simulink model "ES259A_BattVltgCorrln"  (R2013b)
settings: Solver=FixedStepDiscrete  SolverMode=SingleTasking  StartTime=0.0  StopTime=Inf  FixedStep=0.002  RelTol=1e-3
values from neighbouring files (symbols this model uses):
  BattVltgCorrlnAllwdVltgDif = DataDict.Calibration    [ES259A_BattVltgCorrln_DataDict.m]
  BattVltgCorrlnBattLoVltg = DataDict.Calibration    [ES259A_BattVltgCorrln_DataDict.m]
  BattVltgCorrlnBattOverVltg = DataDict.Calibration    [ES259A_BattVltgCorrln_DataDict.m]
  BattVltgCorrlnBattUnderVltg = DataDict.Calibration    [ES259A_BattVltgCorrln_DataDict.m]
  BattVltgCorrlnNtc0x03C0x0440x04CFailStep = DataDict.Calibration    [ES259A_BattVltgCorrln_DataDict.m]
  BattVltgCorrlnNtc0x03C0x0440x04CPassStep = DataDict.Calibration    [ES259A_BattVltgCorrln_DataDict.m]
  BattVltgCorrlnNtc0x03DFailStep = DataDict.Calibration    [ES259A_BattVltgCorrln_DataDict.m]
  BattVltgCorrlnNtc0x03DPassStep = DataDict.Calibration    [ES259A_BattVltgCorrln_DataDict.m]
  BattVltgCorrlnNtc0x0B0FailStep = DataDict.Calibration    [ES259A_BattVltgCorrln_DataDict.m]
  BattVltgCorrlnNtc0x0B0PassStep = DataDict.Calibration    [ES259A_BattVltgCorrln_DataDict.m]
  BattVltgCorrlnNtc0x0B1FailStep = DataDict.Calibration    [ES259A_BattVltgCorrln_DataDict.m]
  BattVltgCorrlnNtc0x0B1PassStep = DataDict.Calibration    [ES259A_BattVltgCorrln_DataDict.m]
  BattVltgCorrlnNtc0x0B5FailStep = DataDict.Calibration    [ES259A_BattVltgCorrln_DataDict.m]
  BattVltgCorrlnNtc0x0B5PassStep = DataDict.Calibration    [ES259A_BattVltgCorrln_DataDict.m]
  BattVltgCorrlnRcvrlBattLoVltg = DataDict.Calibration    [ES259A_BattVltgCorrln_DataDict.m]
  BattVltgCorrlnRcvrlBattOverVltg = DataDict.Calibration    [ES259A_BattVltgCorrln_DataDict.m]
  BattVltgCorrlnRcvrlBattUnderVltg = DataDict.Calibration    [ES259A_BattVltgCorrln_DataDict.m]
  BattVltgCorrlnSysMinVltg = DataDict.ImprtdCal    [ES250A_BattVltg_DataDict.m]    (also in ES259A_BattVltgCorrln_DataDict.m = DataDict.Calibration)
  BattVltgSwdMax = DataDict.Calibration    [ES250A_BattVltg_DataDict.m]
  ELECGLBPRM_STRTUPSTPWRDISCNCTBTESTCMPL_CNT_U08 = DataDict.Constant    [ES999A_ElecGlbPrm_DataDict.m]
  SYSVLTGFLTDUALIVTR_CNT_U08 = DataDict.Constant    [ES259A_BattVltgCorrln_DataDict.m]
undefined symbols (not defined in the file or in its folder): NtcNr1, NtcSts1, SigQlfr1
libraries: simulink x14
(part 1 of 7)
settings Model: Creator=NZG49T  LastModifiedBy=nzg49t
settings SolverCC: AutoInsertRateTranBlk=on  InsertRTBMode=Always
settings DataIOCC: LimitDataPoints=off  SaveFormat=Structure  ReturnWorkspaceOutputs=on
settings OptimizationCC: BlockReduction=off  InlineParams=on  ZeroExternalMemoryAtStartup=off  ZeroInternalMemoryAtStartup=off  OptimizeModelRefInitCode=on  LifeSpan=1
settings DebuggingCC: SignalInfNanChecking=error  SignalRangeChecking=warning  UnderspecifiedInitializationDetection=Simplified  SolverPrmCheckMsg=error  InheritedTsInSrcMsg=error  DiscreteInheritContinuousMsg=error  SingleTaskRateTransMsg=error  TasksWithSamePriorityMsg=error  SigSpecEnsureSampleTimeMsg=error  CheckMatrixSingularityMsg=error  ParameterUnderflowMsg=error  ParameterPrecisionLossMsg=error  ParameterTunabilityLossMsg=error  FixptConstUnderflowMsg=warning  FixptConstOverflowMsg=warning  VectorMatrixConversionMsg=error  SignalLabelMismatchMsg=error  UnconnectedInputMsg=error  UnconnectedOutputMsg=error  UnconnectedLineMsg=error  SFcnCompatibilityMsg=error  UniqueDataStoreMsg=warning  BusObjectLabelMismatch=error  RootOutportRequireBusObject=error  AssertControl=DisableAll  ModelReferenceIOMsg=error  ModelReferenceVersionMismatchMessage=warning  ModelReferenceIOMismatchMessage=error  ModelReferenceCSMismatchMessage=warning  ModelReferenceDataLoggingMessage=error  StateNameClashWarn=warning  StrictBusMsg=ErrorOnBusTreatedAsVector  NonBusSignalsTreatedAsBus=error  SFUnexpectedBacktrackingDiag=error  SFInvalidInputDataAccessInChartInitDiag=error  SFNoUnconditionalDefaultTransitionDiag=error  SFTransitionOutsideNaturalParentDiag=error  SFUnconditionalTransitionShadowingDiag=error  SFUndirectedBroadcastEventsDiag=error
settings ModelReferenceCC: ModelReferenceNumInstancesAllowed=Single
settings RTWCC: SystemTargetFile=autosar.tlc  GenCodeOnly=on  TemplateMakefile=ert_default_tmf  Description=AUTOSAR  GenerateReport=on  ProcessScript=autosar_make_rtw_hook  LaunchReport=on
settings CodeAppCC: GenerateComments=off  IgnoreCustomStorageClasses=off  CustomSymbolStrType=$N$R$M  CustomSymbolStrBlkIO=$N$M  SimulinkBlockComments=off
settings STFCustomTargetCC: ParMdlRefBuildCompliant=on  CompOptLevelCompliant=on  IncludeMdlTerminateFcn=off  CombineOutputUpdateFcns=on  SuppressErrorStatus=on  ERTFirstTimeCompliant=on  ERTCustomFileBanners=on  SupportNonFinite=off  SupportComplex=off  SupportContinuousTime=off  SupportNonInlinedSFcns=off  MATLABClassNameForMDSCustomization=Simulink.SoftwareTarget.ERTCustomization  AutosarCompliant=on  GRTInterface=off  SystemTargetFile=autosar.tlc
settings ERTTargetCC: CodeReplacementLibrary=ANSI_C  ConcurrentExecutionCompliant=off  IncludeMdlTerminateFcn=off  SuppressErrorStatus=on  SupportNonFinite=off  SupportComplex=off  ModelStepFunctionPrototypeControlCompliant=off  CPPClassGenCompliant=off  AutosarCompliant=on  InlinedParameterPlacement=NonHierarchical  ERTCustomFileTemplate=example_file_process.tlc  EnableUserReplacementTypes=on

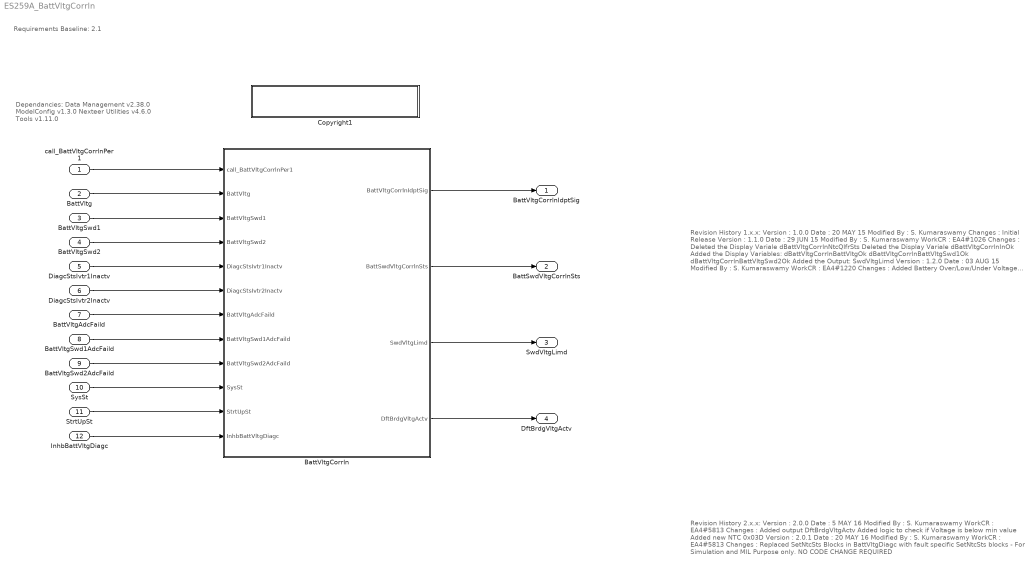
== system ES259A_BattVltgCorrln ==
  note: Revision History 1.x.x:
      |
      | Version		:	1.0.0
      | Date 		:	20 MAY 15
      | Modified By	:	S. Kumaraswamy
      | Changes		:	Initial Release
      |
      | Version		:	1.1.0
      | Date 		:	29 JUN 15
      | Modified By	:	S. Kumaraswamy
      | WorkCR 	:	EA4#1026
      | Changes		:	Deleted the Display Variale dBattVltgCorrlnNtcQlfrSts
      | 				Deleted the Display Variale dBattVltgCorrlnInOk
      | 				Added the Display Variables:
      | 					dBattVltgCorrlnBattVltgOk
      | 					dBattVltgCorrlnBattVltgSwd1Ok
      | 					dBattVltgCorrlnBattVltgSwd2Ok
      | 				Added the Output:
      | 					SwdVltgLimd
      |
      | Version		:	1.2.0
      | Date 		:	03 AUG 15
      | Modified By	:	S. Kumaraswamy
      | WorkCR 	:	EA4#1220
      | Changes		:	Added Battery Over/Low/Under Voltage Diagnostics
      | 				Added input signal InhbBattVltgDiagc
      |
      | Version		:	1.3.0
      | Date 		:	05 OCT 15
      | Modified By	:	S. Kumaraswamy
      | WorkCR 	:	EA4#1220
      | Changes		:	In .m file, InhbBattVltgDiagc.EngInit = 1 changed to InhbBattVltgDiagc.EngInit = 0
      |
      |
      | Version		:	1.4.0
      | Date 		:	18 MAR 16
      | Modified By	:	 Praveen Devaraj / Muragesh Asundi (KPIT)
      | WorkCR 	:	 EA4#4317
      | Changes		:	As per the new requirement three AdcFaild inputs and logic for these are added
      | 				The data store blocks "A" which was used for simultaion purpose  has been removed and
      |                              path where it was present earlier has been highlighted. This change has no impact on code.
  note: Dependancies:
      |
      | 	Data Management v2.38.0
      | 	ModelConfig v1.3.0
      |   	Nexteer Utilities v4.6.0
      | 	Tools v1.11.0
  note: Requirements Baseline: 2.1
  note: Revision History 2.x.x:
      |
      | Version		:	2.0.0
      | Date 		:	5 MAY 16
      | Modified By	:	S. Kumaraswamy
      | WorkCR		:	EA4#5813
      | Changes		:	Added output DftBrdgVltgActv
      | 				Added logic to check if Voltage is below min value
      | 				Added new NTC 0x03D
      |
      | Version		:	2.0.1
      | Date 		:	20 MAY 16
      | Modified By	:	S. Kumaraswamy
      | WorkCR		:	EA4#5813
      | Changes		:	Replaced SetNtcSts Blocks in BattVltgDiagc with fault specific SetNtcSts blocks - For Simulation and MIL Purpose only.
      | 				NO CODE CHANGE REQUIRED
  call_BattVltgCorrlnPer1 : Inport
  BattVltg : Inport  RequirementInfo={} %GIDa_9ae0aaec_9b84_4091_a1e8_9e8c099ef51a  Port=2
  BattVltgSwd1 : Inport  RequirementInfo={} %GIDa_9c84e353_52aa_468c_bc43_36e071f85c19  Port=3
  BattVltgSwd2 : Inport  RequirementInfo={} %GIDa_90dc59e4_2ab9_47b5_8004_0d538e7055af  Port=4
  DiagcStsIvtr1Inactv : Inport  RequirementInfo={} %GIDa_f8e15c53_514a_4131_9fe2_6d94161aaaeb  Port=5  OutDataTypeStr=boolean
  DiagcStsIvtr2Inactv : Inport  RequirementInfo={} %GIDa_3b2c6370_c505_4ccf_a518_ab0f64efa1b9  Port=6  OutDataTypeStr=boolean
  BattVltgAdcFaild : Inport  RequirementInfo={} %GIDa_ee986134_339a_4ec6_a7d6_a1f80f3bff1f  Port=7
  BattVltgSwd1AdcFaild : Inport  RequirementInfo={} %GIDa_e9391629_cfd6_4a15_93e9_ed299c660fed  Port=8
  BattVltgSwd2AdcFaild : Inport  RequirementInfo={} %GIDa_fb77af98_ead1_4424_a254_76551fbf463c  Port=9
  SysSt : Inport  RequirementInfo={} %GIDa_3959cee0_aa32_4855_b980_1d0b1d7c6b22  Port=10
  StrtUpSt : Inport  RequirementInfo={} %GIDa_35521d03_63d6_4c56_948e_5f048d51783f  Port=11
  InhbBattVltgDiagc : Inport  RequirementInfo={} %GIDa_d10198bb_1424_48c8_be8f_3c2405f9ced0  Port=12
  BattVltgCorrln : Subsystem
  Copyright1 : Subsystem  Description=|  mask(Copyright Information){none=on}
      | Copyright info block.                                               
      |                                                                     
      | Place copyright information at the top of every subsystem in design.
      mask prompts: none "No parameters"
      mask help: Place copyright information at the top of every subsystem in design.
      mask Display:
      | NxtrConf = 'Nexteer Confidential';
      | 
      | sys = bdroot; %handle for the current model ("system")
      | first = get_param(sys,'Created');
      | if(isempty(first))
      |     first = datestr(now,'yyyy');
      | else
      |     first = first(end-3:end);  %year is last four digits
      | end
      | 
      | last = get_param(sys,'LastModifiedDate');
      | if isempty(last)
      |     last = datestr(now,'yyyy');
      | else
      |     last = last(end-3:end);
      | end
      | 
      | if strcmp(first,last)
      |     fprintf('%s\nCopyright  %s Nexteer',NxtrConf,first);
      | else
      |     fprintf('%s\n%s%s-%s Nexteer',NxtrConf,char(169),first,last);
      | end
  BattVltgCorrlnIdptSig : Outport  RequirementInfo={} %GIDa_aec574ca_5fa5_4de5_85a2_6855dbe6e557
  BattSwdVltgCorrlnSts : Outport  RequirementInfo={} %GIDa_7fe09802_8610_498d_8b99_46ac352eb16c  Port=2
  SwdVltgLimd : Outport  RequirementInfo={} %GIDa_1e8b1924_aadb_4bf8_9d90_544eb8aa499f  Port=3  InitialOutput=0
  DftBrdgVltgActv : Outport  RequirementInfo={} %GIDa_446ef28e_3990_43bd_ac3d_a3cd0694cd31  Port=4  InitialOutput=0
  wires:
  BattVltgCorrln/3(SwdVltgLimd) -> SwdVltgLimd/1
  BattVltgCorrln/4(DftBrdgVltgActv) -> DftBrdgVltgActv/1
  BattVltgCorrln/2(BattSwdVltgCorrlnSts) -> BattSwdVltgCorrlnSts/1
  BattVltgCorrln/1(BattVltgCorrlnIdptSig) -> BattVltgCorrlnIdptSig/1
  BattVltgSwd2AdcFaild/1 -> BattVltgCorrln/9(BattVltgSwd2AdcFaild)
  BattVltgSwd1AdcFaild/1 -> BattVltgCorrln/8(BattVltgSwd1AdcFaild)
  SysSt/1 -> BattVltgCorrln/10(SysSt)
  StrtUpSt/1 -> BattVltgCorrln/11(StrtUpSt)
  BattVltgAdcFaild/1 -> BattVltgCorrln/7(BattVltgAdcFaild)
  InhbBattVltgDiagc/1 -> BattVltgCorrln/12(InhbBattVltgDiagc)
  DiagcStsIvtr2Inactv/1 -> BattVltgCorrln/6(DiagcStsIvtr2Inactv)
  DiagcStsIvtr1Inactv/1 -> BattVltgCorrln/5(DiagcStsIvtr1Inactv)
  BattVltgSwd2/1 -> BattVltgCorrln/4(BattVltgSwd2)
  BattVltgSwd1/1 -> BattVltgCorrln/3(BattVltgSwd1)
  BattVltg/1 -> BattVltgCorrln/2(BattVltg)
  call_BattVltgCorrlnPer1/1 -> BattVltgCorrln/1(call_BattVltgCorrlnPer1)

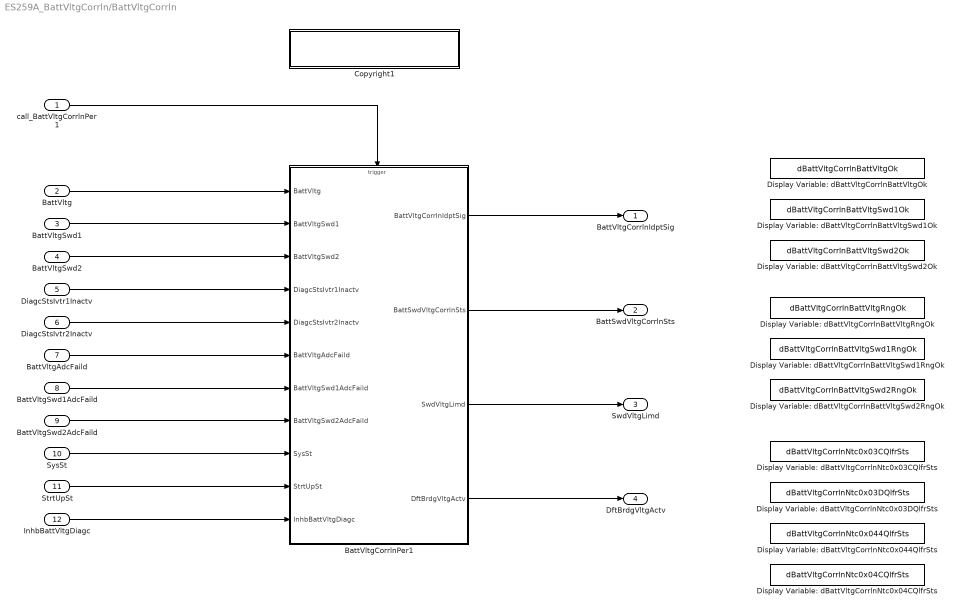
== system ES259A_BattVltgCorrln/BattVltgCorrln ==
  call_BattVltgCorrlnPer1 : Inport
  BattVltg : Inport  RequirementInfo={} %GIDa_f126ed04_401f_4bfa_94c3_1fe23454bc4c  Port=2
  BattVltgSwd1 : Inport  RequirementInfo={} %GIDa_f8722f2f_fc01_4116_8ff7_50c79c8e6a7f  Port=3
  BattVltgSwd2 : Inport  RequirementInfo={} %GIDa_5334dfc7_2389_4d4c_8517_7c435322b8bc  Port=4
  DiagcStsIvtr1Inactv : Inport  RequirementInfo={} %GIDa_58bb2539_964f_4ead_88ba_e608502c7aa6  Port=5  OutDataTypeStr=boolean
  DiagcStsIvtr2Inactv : Inport  RequirementInfo={} %GIDa_c153f17a_f8b8_4fc8_b318_6e5ea34530c6  Port=6  OutDataTypeStr=boolean
  BattVltgAdcFaild : Inport  RequirementInfo={} %GIDa_9c98f6c9_a87c_456c_aacd_351e973b6c42  Port=7
  BattVltgSwd1AdcFaild : Inport  RequirementInfo={} %GIDa_4b863112_3bcd_4930_bdb0_947e74b9095a  Port=8
  BattVltgSwd2AdcFaild : Inport  RequirementInfo={} %GIDa_42ec5868_b1c2_41ea_8fe7_d58ef520f1c8  Port=9
  SysSt : Inport  RequirementInfo={} %GIDa_f147f53a_7a4f_488c_80dd_1465aa705151  Port=10
  StrtUpSt : Inport  RequirementInfo={} %GIDa_988f5f6c_af97_4280_8e31_9d7a0d15c864  Port=11
  InhbBattVltgDiagc : Inport  RequirementInfo={} %GIDa_08e5665b_47e5_442a_9c58_120194cd1682  Port=12
  BattVltgCorrlnPer1 : Subsystem
  Copyright1 : Subsystem  Description=|  mask(Copyright Information){none=on}
      | Copyright info block.                                               
      |                                                                     
      | Place copyright information at the top of every subsystem in design.
      mask prompts: none "No parameters"
      mask help: Place copyright information at the top of every subsystem in design.
      mask Display:
      | NxtrConf = 'Nexteer Confidential';
      | 
      | sys = bdroot; %handle for the current model ("system")
      | first = get_param(sys,'Created');
      | if(isempty(first))
      |     first = datestr(now,'yyyy');
      | else
      |     first = first(end-3:end);  %year is last four digits
      | end
      | 
      | last = get_param(sys,'LastModifiedDate');
      | if isempty(last)
      |     last = datestr(now,'yyyy');
      | else
      |     last = last(end-3:end);
      | end
      | 
      | if strcmp(first,last)
      |     fprintf('%s\nCopyright  %s Nexteer',NxtrConf,first);
      | else
      |     fprintf('%s\n%s%s-%s Nexteer',NxtrConf,char(169),first,last);
      | end
  Display Variable: dBattVltgCorrlnBattVltgOk : DataStoreMemory  DataStoreName=dBattVltgCorrlnBattVltgOk  OutDataTypeStr=uint8  StateMustResolveToSignalObject=on
  Display Variable: dBattVltgCorrlnBattVltgRngOk : DataStoreMemory  DataStoreName=dBattVltgCorrlnBattVltgRngOk  OutDataTypeStr=uint8  StateMustResolveToSignalObject=on
  Display Variable: dBattVltgCorrlnBattVltgSwd1Ok : DataStoreMemory  DataStoreName=dBattVltgCorrlnBattVltgSwd1Ok  OutDataTypeStr=uint8  StateMustResolveToSignalObject=on
  Display Variable: dBattVltgCorrlnBattVltgSwd1RngOk : DataStoreMemory  DataStoreName=dBattVltgCorrlnBattVltgSwd1RngOk  OutDataTypeStr=uint8  StateMustResolveToSignalObject=on
  Display Variable: dBattVltgCorrlnBattVltgSwd2Ok : DataStoreMemory  DataStoreName=dBattVltgCorrlnBattVltgSwd2Ok  OutDataTypeStr=uint8  StateMustResolveToSignalObject=on
  Display Variable: dBattVltgCorrlnBattVltgSwd2RngOk : DataStoreMemory  DataStoreName=dBattVltgCorrlnBattVltgSwd2RngOk  OutDataTypeStr=uint8  StateMustResolveToSignalObject=on
  Display Variable: dBattVltgCorrlnNtc0x03CQlfrSts : DataStoreMemory  DataStoreName=dBattVltgCorrlnNtc0x03CQlfrSts  OutDataTypeStr=Enum: SigQlfr1  StateMustResolveToSignalObject=on
  Display Variable: dBattVltgCorrlnNtc0x03DQlfrSts : DataStoreMemory  DataStoreName=dBattVltgCorrlnNtc0x03DQlfrSts  OutDataTypeStr=Enum: SigQlfr1  StateMustResolveToSignalObject=on
  Display Variable: dBattVltgCorrlnNtc0x044QlfrSts : DataStoreMemory  DataStoreName=dBattVltgCorrlnNtc0x044QlfrSts  OutDataTypeStr=Enum: SigQlfr1  StateMustResolveToSignalObject=on
  Display Variable: dBattVltgCorrlnNtc0x04CQlfrSts : DataStoreMemory  DataStoreName=dBattVltgCorrlnNtc0x04CQlfrSts  OutDataTypeStr=Enum: SigQlfr1  StateMustResolveToSignalObject=on
  BattVltgCorrlnIdptSig : Outport  RequirementInfo={} %GIDa_5ee6736b_40f2_4c1a_b85a_65eebdb316c2
  BattSwdVltgCorrlnSts : Outport  RequirementInfo={} %GIDa_bd9620c8_c3f8_451b_a2d9_6d23915e6e1a  Port=2
  SwdVltgLimd : Outport  RequirementInfo={} %GIDa_4a11c4bf_f696_4399_ae2f_3380c1da49be  Port=3  InitialOutput=0
  DftBrdgVltgActv : Outport  RequirementInfo={} %GIDa_5c9b650e_dee9_4d60_997e_bde7a993e084  Port=4  InitialOutput=0
  wires:
  BattVltg/1 -> BattVltgCorrlnPer1/1(BattVltg)
  BattVltgSwd1/1 -> BattVltgCorrlnPer1/2(BattVltgSwd1)
  BattVltgSwd2/1 -> BattVltgCorrlnPer1/3(BattVltgSwd2)
  BattVltgCorrlnPer1/1(BattVltgCorrlnIdptSig) -> BattVltgCorrlnIdptSig/1
  DiagcStsIvtr2Inactv/1 -> BattVltgCorrlnPer1/5(DiagcStsIvtr2Inactv)
  StrtUpSt/1 -> BattVltgCorrlnPer1/10(StrtUpSt)
  SysSt/1 -> BattVltgCorrlnPer1/9(SysSt)
  DiagcStsIvtr1Inactv/1 -> BattVltgCorrlnPer1/4(DiagcStsIvtr1Inactv)
  call_BattVltgCorrlnPer1/1 -> BattVltgCorrlnPer1/Trigger
  BattVltgCorrlnPer1/2(BattSwdVltgCorrlnSts) -> BattSwdVltgCorrlnSts/1
  BattVltgCorrlnPer1/3(SwdVltgLimd) -> SwdVltgLimd/1
  InhbBattVltgDiagc/1 -> BattVltgCorrlnPer1/11(InhbBattVltgDiagc)
  BattVltgSwd2AdcFaild/1 -> BattVltgCorrlnPer1/8(BattVltgSwd2AdcFaild)
  BattVltgSwd1AdcFaild/1 -> BattVltgCorrlnPer1/7(BattVltgSwd1AdcFaild)
  BattVltgAdcFaild/1 -> BattVltgCorrlnPer1/6(BattVltgAdcFaild)
  BattVltgCorrlnPer1/4(DftBrdgVltgActv) -> DftBrdgVltgActv/1

== system ES259A_BattVltgCorrln/Copyright1 ==

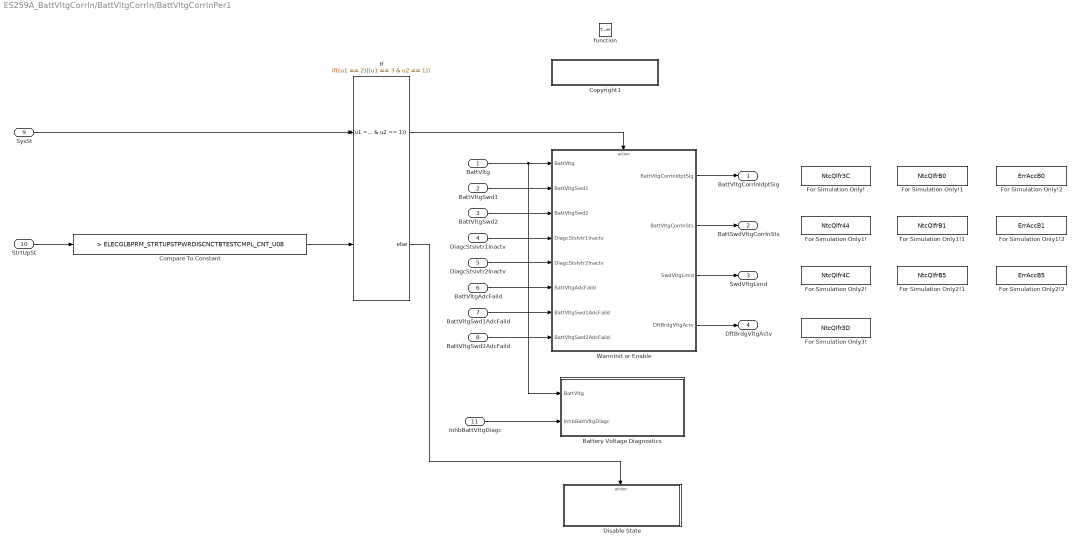
== system ES259A_BattVltgCorrln/BattVltgCorrln/BattVltgCorrlnPer1 ==
  BattVltg : Inport
  BattVltgSwd1 : Inport  Port=2  OutDataTypeStr=single
  BattVltgSwd2 : Inport  Port=3  OutDataTypeStr=single
  DiagcStsIvtr1Inactv : Inport  Port=4  OutDataTypeStr=boolean
  DiagcStsIvtr2Inactv : Inport  Port=5  OutDataTypeStr=boolean
  BattVltgAdcFaild : Inport  Port=6
  BattVltgSwd1AdcFaild : Inport  Port=7
  BattVltgSwd2AdcFaild : Inport  Port=8
  SysSt : Inport  Port=9
  StrtUpSt : Inport  Port=10
  InhbBattVltgDiagc : Inport  Port=11  OutDataTypeStr=boolean
  function : TriggerPort  TriggerType=function-call
  Battery Voltage Diagnostics : Subsystem  RequirementInfo="{'linktype_rmi_doors' '0000cf46 (/ESG Group/FDD Module Requirements/EA4 Specific/ES259A_BattVltgCorrln)' '#ES259A_171' 'true' 'REQ:  ES259A_171' '' ; 'linktype_rmi_doors' '0000cf46 (/ESG Group/FDD Module Requirements/EA4 Specific/ES259A_BattVltgCorrln)' '#ES259A_172' 'true' 'REQ:  ES259A_172' '' ; 'linktype_rmi_doors' '0000cf46 (/ESG Group/FDD Module Requirements/EA4 Specific/ES259A_BattVltgCorrln)' '#ES259A_174' 'true' 'REQ:  ES259A_174' '' ; 'linktype_rmi_doors' '0000cf46 (/ESG Group/FDD Module Requirements/EA4 Specific/ES259A_BattVltgCorrln)' '#ES259A_175' 'true' 'REQ:  ES259A_175' '' ; 'linktype_rmi_doors' '0000cf46 (/ESG Group/FDD Module Requirements/EA4 Specific/ES259A_BattVltgCorrln)' '#ES259A_177' 'true' 'REQ:  ES259A_177' '' ; 'linktype_rmi_doors' '0000cf46 (/ESG Group/FDD Module Requirements/EA4 Specific/ES259A_BattVltgCorrln)' '#ES259A_178' 'true' 'REQ:  ES259A_178' '' ; 'linktype_rmi_doors' '0000cf46 (/ESG Group/FDD Module Requirements/EA4 Specific/ES259A_BattVltgCorrln)' '#ES259A_180' 'true' 'REQ:  ES259A_180' '' ; 'linktype_rmi_doors' '0000cf46 (/ESG Group/FDD Module Requirements/EA4 Specific/ES259A_BattVltgCorrln)' '#ES259A_182' 'true' 'REQ:  ES259A_182' '' ; 'linktype_rmi_doors' '0000cf46 (/ESG Group/FDD Module Requirements/EA4 Specific/ES259A_BattVltgCorrln)' '#ES259A_183' 'true' 'REQ:  ES259A_183' '' ; 'linktype_rmi_doors' '0000cf46 (/ESG Group/FDD Module Requirements/EA4 Specific/ES259A_BattVltgCorrln)' '#ES259A_184' 'true' 'REQ:  ES259A_184' '' ; 'linktype_rmi_doors' '0000cf46 (/ESG Group/FDD Module Requirements/EA4 Specific/ES259A_BattVltgCorrln)' '#ES259A_186' 'true' 'REQ:  ES259A_186' '' ; 'linktype_rmi_doors' '0000cf46 (/ESG Group/FDD Module Requirements/EA4 Specific/ES259A_BattVltgCorrln)' '#ES259A_188' 'true' 'REQ:  ES259A_188' '' } %GIDa_c0de6c2c_8549_4a12_9f62_e9a08cdbf394"
  Compare To Constant : simulink/Logic and Bit Operations/Compare To Constant  relop=>  const=ELECGLBPRM_STRTUPSTPWRDISCNCTBTESTCMPL_CNT_U08  OutDataTypeStr=uint8
  Copyright1 : Subsystem  Description=|  mask(Copyright Information){none=on}
      | Copyright info block.                                               
      |                                                                     
      | Place copyright information at the top of every subsystem in design.
      mask prompts: none "No parameters"
      mask help: Place copyright information at the top of every subsystem in design.
      mask Display:
      | NxtrConf = 'Nexteer Confidential';
      | 
      | sys = bdroot; %handle for the current model ("system")
      | first = get_param(sys,'Created');
      | if(isempty(first))
      |     first = datestr(now,'yyyy');
      | else
      |     first = first(end-3:end);  %year is last four digits
      | end
      | 
      | last = get_param(sys,'LastModifiedDate');
      | if isempty(last)
      |     last = datestr(now,'yyyy');
      | else
      |     last = last(end-3:end);
      | end
      | 
      | if strcmp(first,last)
      |     fprintf('%s\nCopyright  %s Nexteer',NxtrConf,first);
      | else
      |     fprintf('%s\n%s%s-%s Nexteer',NxtrConf,char(169),first,last);
      | end
  Disable State : Subsystem  TreatAsAtomicUnit=on
  For Simulation Only! : DataStoreMemory  DataStoreName=NtcQlfr3C
  For Simulation Only!1 : DataStoreMemory  DataStoreName=NtcQlfrB0
  For Simulation Only!2 : DataStoreMemory  DataStoreName=ErrAccB0  OutDataTypeStr=int16
  For Simulation Only1! : DataStoreMemory  DataStoreName=NtcQlfr44
  For Simulation Only1!1 : DataStoreMemory  DataStoreName=NtcQlfrB1
  For Simulation Only1!2 : DataStoreMemory  DataStoreName=ErrAccB1  OutDataTypeStr=int16
  For Simulation Only2! : DataStoreMemory  DataStoreName=NtcQlfr4C
  For Simulation Only2!1 : DataStoreMemory  DataStoreName=NtcQlfrB5
  For Simulation Only2!2 : DataStoreMemory  DataStoreName=ErrAccB5  OutDataTypeStr=int16
  For Simulation Only3! : DataStoreMemory  DataStoreName=NtcQlfr3D
  If : If  NumInputs=2  IfExpression=(u1 == 2)|(u1 == 3 & u2 == 1)
  WarmInit or Enable : Subsystem  TreatAsAtomicUnit=on
  BattVltgCorrlnIdptSig : Outport
  BattSwdVltgCorrlnSts : Outport  RequirementInfo={} %GIDa_3ad73624_6641_44da_a28f_9988e11678b5  Port=2  InitialOutput=0
  SwdVltgLimd : Outport  RequirementInfo={} %GIDa_5f7e1f7f_e198_46a1_a24d_58ddfd5d3a89  Port=3  InitialOutput=0
  DftBrdgVltgActv : Outport  RequirementInfo={} %GIDa_cedb6ec7_b563_4bca_a7d5_9398ac57a3e7  Port=4  InitialOutput=0
  wires:
  If/2 -> Disable State/Action
  If/1 -> WarmInit or Enable/Action
  BattVltgSwd1/1 -> WarmInit or Enable/2(BattVltgSwd1)
  BattVltgSwd2/1 -> WarmInit or Enable/3(BattVltgSwd2)
  DiagcStsIvtr1Inactv/1 -> WarmInit or Enable/4(DiagcStsIvtr1Inactv)
  DiagcStsIvtr2Inactv/1 -> WarmInit or Enable/5(DiagcStsIvtr2Inactv)
  WarmInit or Enable/1(BattVltgCorrlnIdptSig) -> BattVltgCorrlnIdptSig/1
  WarmInit or Enable/2(BattVltgCorrlnSts) -> BattSwdVltgCorrlnSts/1
  StrtUpSt/1 -> Compare To Constant/1
  Compare To Constant/1 -> If/2
  SysSt/1 -> If/1
  WarmInit or Enable/3(SwdVltgLimd) -> SwdVltgLimd/1
  InhbBattVltgDiagc/1 -> Battery Voltage Diagnostics/2(InhbBattVltgDiagc)
  BattVltg/1 -> Battery Voltage Diagnostics/1(BattVltg), WarmInit or Enable/1(BattVltg)
  BattVltgAdcFaild/1 -> WarmInit or Enable/6(BattVltgAdcFaild)
  BattVltgSwd2AdcFaild/1 -> WarmInit or Enable/8(BattVltgSwd2AdcFaild)
  BattVltgSwd1AdcFaild/1 -> WarmInit or Enable/7(BattVltgSwd1AdcFaild)
  WarmInit or Enable/4(DftBrdgVltgActv) -> DftBrdgVltgActv/1

== system ES259A_BattVltgCorrln/BattVltgCorrln/Copyright1 ==

== system ES259A_BattVltgCorrln/BattVltgCorrln/BattVltgCorrlnPer1/Battery Voltage Diagnostics ==
  BattVltg : Inport
  InhbBattVltgDiagc : Inport  Port=2
  Copyright1 : Subsystem  Description=|  mask(Copyright Information){none=on}
      | Copyright info block.                                               
      |                                                                     
      | Place copyright information at the top of every subsystem in design.
      mask prompts: none "No parameters"
      mask help: Place copyright information at the top of every subsystem in design.
      mask Display:
      | NxtrConf = 'Nexteer Confidential';
      | 
      | sys = bdroot; %handle for the current model ("system")
      | first = get_param(sys,'Created');
      | if(isempty(first))
      |     first = datestr(now,'yyyy');
      | else
      |     first = first(end-3:end);  %year is last four digits
      | end
      | 
      | last = get_param(sys,'LastModifiedDate');
      | if isempty(last)
      |     last = datestr(now,'yyyy');
      | else
      |     last = last(end-3:end);
      | end
      | 
      | if strcmp(first,last)
      |     fprintf('%s\nCopyright  %s Nexteer',NxtrConf,first);
      | else
      |     fprintf('%s\n%s%s-%s Nexteer',NxtrConf,char(169),first,last);
      | end
  If : If  IfExpression=u1 == 0
  Inhibition Off : Subsystem  RequirementInfo={} %GIDa_f00050e4_548b_4aa2_8c05_f34bff13809e  TreatAsAtomicUnit=on
  Inhibition On : Subsystem  TreatAsAtomicUnit=on
  wires:
  InhbBattVltgDiagc/1 -> If/1
  If/1 -> Inhibition Off/Action
  If/2 -> Inhibition On/Action
  BattVltg/1 -> Inhibition Off/1(BattVltg)

== system ES259A_BattVltgCorrln/BattVltgCorrln/BattVltgCorrlnPer1/Copyright1 ==

== system ES259A_BattVltgCorrln/BattVltgCorrln/BattVltgCorrlnPer1/Disable State ==
  Action Port : ActionPort  ActionType=else
  Copyright1 : Subsystem  Description=|  mask(Copyright Information){none=on}
      | Copyright info block.                                               
      |                                                                     
      | Place copyright information at the top of every subsystem in design.
      mask prompts: none "No parameters"
      mask help: Place copyright information at the top of every subsystem in design.
      mask Display:
      | NxtrConf = 'Nexteer Confidential';
      | 
      | sys = bdroot; %handle for the current model ("system")
      | first = get_param(sys,'Created');
      | if(isempty(first))
      |     first = datestr(now,'yyyy');
      | else
      |     first = first(end-3:end);  %year is last four digits
      | end
      | 
      | last = get_param(sys,'LastModifiedDate');
      | if isempty(last)
      |     last = datestr(now,'yyyy');
      | else
      |     last = last(end-3:end);
      | end
      | 
      | if strcmp(first,last)
      |     fprintf('%s\nCopyright  %s Nexteer',NxtrConf,first);
      | else
      |     fprintf('%s\n%s%s-%s Nexteer',NxtrConf,char(169),first,last);
      | end

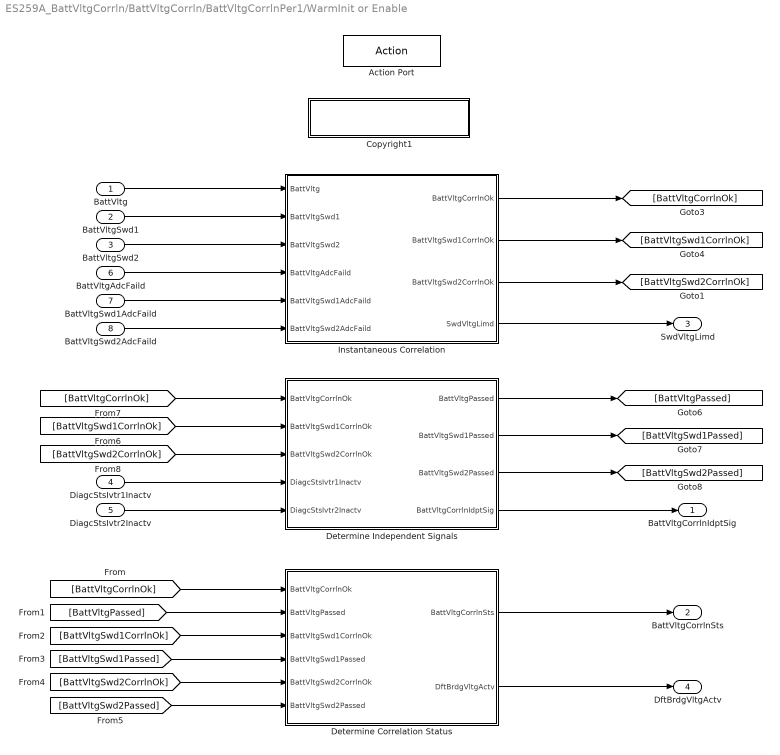
== system ES259A_BattVltgCorrln/BattVltgCorrln/BattVltgCorrlnPer1/WarmInit or Enable ==
  BattVltg : Inport
  BattVltgSwd1 : Inport  Port=2
  BattVltgSwd2 : Inport  Port=3
  DiagcStsIvtr1Inactv : Inport  RequirementInfo={} %GIDa_ea0b0d04_c797_446a_8c23_09b9fa319238  Port=4
  DiagcStsIvtr2Inactv : Inport  RequirementInfo={} %GIDa_940c0479_90c1_4645_b5ad_7886f1cabd09  Port=5
  BattVltgAdcFaild : Inport  Port=6
  BattVltgSwd1AdcFaild : Inport  Port=7
  BattVltgSwd2AdcFaild : Inport  Port=8
  Action Port : ActionPort  ActionType=then
  Copyright1 : Subsystem  Description=|  mask(Copyright Information){none=on}
      | Copyright info block.                                               
      |                                                                     
      | Place copyright information at the top of every subsystem in design.
      mask prompts: none "No parameters"
      mask help: Place copyright information at the top of every subsystem in design.
      mask Display:
      | NxtrConf = 'Nexteer Confidential';
      | 
      | sys = bdroot; %handle for the current model ("system")
      | first = get_param(sys,'Created');
      | if(isempty(first))
      |     first = datestr(now,'yyyy');
      | else
      |     first = first(end-3:end);  %year is last four digits
      | end
      | 
      | last = get_param(sys,'LastModifiedDate');
      | if isempty(last)
      |     last = datestr(now,'yyyy');
      | else
      |     last = last(end-3:end);
      | end
      | 
      | if strcmp(first,last)
      |     fprintf('%s\nCopyright  %s Nexteer',NxtrConf,first);
      | else
      |     fprintf('%s\n%s%s-%s Nexteer',NxtrConf,char(169),first,last);
      | end
  Determine Correlation Status : Subsystem  RequirementInfo="{'linktype_rmi_doors' '0000cf46 (/ESG Group/FDD Module Requirements/EA4 Specific/ES259A_BattVltgCorrln)' '#ES259A_16' 'true' 'REQ:  ES259A_16' '' ; 'linktype_rmi_doors' '0000cf46 (/ESG Group/FDD Module Requirements/EA4 Specific/ES259A_BattVltgCorrln)' '#ES259A_76' 'true' 'REQ:  ES259A_76' '' ; 'linktype_rmi_doors' '0000cf46 (/ESG Group/FDD Module Requirements/EA4 Specific/ES259A_BattVltgCorrln)' '#ES259A_75' 'true' 'REQ:  ES259A_75' '' ; 'linktype_rmi_doors' '0000cf46 (/ESG Group/FDD Module Requirements/EA4 Specific/ES259A_BattVltgCorrln)' '#ES259A_225' 'true' 'REQ:  ES259A_225' '' ; 'linktype_rmi_doors' '0000cf46 (/ESG Group/FDD Module Requirements/EA4 Specific/ES259A_BattVltgCorrln)' '#ES259A_83' 'true' 'REQ:  ES259A_83' '' ; 'linktype_rmi_doors' '0000cf46 (/ESG Group/FDD Module Requirements/EA4 Specific/ES259A_BattVltgCorrln)' '#ES259A_226' 'true' 'REQ:  ES259A_226' '' ; 'linktype_rmi_doors' '0000cf46 (/ESG Group/FDD Module Requirements/EA4 Specific/ES259A_BattVltgCorrln)' '#ES259A_84' 'true' 'REQ:  ES259A_84' '' ; 'linktype_rmi_doors' '0000cf46 (/ESG Group/FDD Module Requirements/EA4 Specific/ES259A_BattVltgCorrln)' '#ES259A_212' 'true' 'REQ:  ES259A_212' '' ; 'linktype_rmi_doors' '0000cf46 (/ESG Group/FDD Module Requirements/EA4 Specific/ES259A_BattVltgCorrln)' '#ES259A_213' 'true' 'REQ:  ES259A_213' '' } %GIDa_1d063a71_29a3_4568_848e_95b2eb318e53"  Priority=3
  Determine Independent Signals : Subsystem  RequirementInfo="{'linktype_rmi_doors' '0000cf46 (/ESG Group/FDD Module Requirements/EA4 Specific/ES259A_BattVltgCorrln)' '#ES259A_74' 'true' 'REQ:  ES259A_74' '' ; 'linktype_rmi_doors' '0000cf46 (/ESG Group/FDD Module Requirements/EA4 Specific/ES259A_BattVltgCorrln)' '#ES259A_78' 'true' 'REQ:  ES259A_78' '' ; 'linktype_rmi_doors' '0000cf46 (/ESG Group/FDD Module Requirements/EA4 Specific/ES259A_BattVltgCorrln)' '#ES259A_80' 'true' 'REQ:  ES259A_80' '' ; 'linktype_rmi_doors' '0000cf46 (/ESG Group/FDD Module Requirements/EA4 Specific/ES259A_BattVltgCorrln)' '#ES259A_73' 'true' 'REQ:  ES259A_73' '' ; 'linktype_rmi_doors' '0000cf46 (/ESG Group/FDD Module Requirements/EA4 Specific/ES259A_BattVltgCorrln)' '#ES259A_81' 'true' 'REQ:  ES259A_81' '' ; 'linktype_rmi_doors' '0000cf46 (/ESG Group/FDD Module Requirements/EA4 Specific/ES259A_BattVltgCorrln)' '#ES259A_139' 'true' 'REQ:  ES259A_139' '' ; 'linktype_rmi_doors' '0000cf46 (/ESG Group/FDD Module Requirements/EA4 Specific/ES259A_BattVltgCorrln)' '#ES259A_140' 'true' 'REQ:  ES259A_140' '' ; 'linktype_rmi_doors' '0000cf46 (/ESG Group/FDD Module Requirements/EA4 Specific/ES259A_BattVltgCorrln)' '#ES259A_141' 'true' 'REQ:  ES259A_141' '' } %GIDa_e656156f_a587_48cc_aa93_4cda59f129ee"  Priority=2
  Instantaneous Correlation : Subsystem  RequirementInfo={} %GIDa_7336d5d0_030f_4090_9dff_c7c935f04c3f  Priority=1
  BattVltgCorrlnIdptSig : Outport  RequirementInfo={} %GIDa_3db734da_8cc6_4e79_92d5_f66bd044e35c  OutDataTypeStr=uint8
  BattVltgCorrlnSts : Outport  RequirementInfo={} %GIDa_20e3ae50_7c15_4536_8fae_c5151833c420  Port=2  OutDataTypeStr=uint8
  SwdVltgLimd : Outport  RequirementInfo={} %GIDa_a517539c_da0e_494d_8ac6_5179314f6f53  Port=3  OutDataTypeStr=boolean
  DftBrdgVltgActv : Outport  Port=4
  wires:
  BattVltg/1 -> Instantaneous Correlation/1(BattVltg)
  BattVltgSwd1/1 -> Instantaneous Correlation/2(BattVltgSwd1)
  BattVltgSwd2/1 -> Instantaneous Correlation/3(BattVltgSwd2)
  Instantaneous Correlation/1(BattVltgCorrlnOk) -> [BattVltgCorrlnOk]
  Instantaneous Correlation/2(BattVltgSwd1CorrlnOk) -> [BattVltgSwd1CorrlnOk]
  [BattVltgCorrlnOk] -> Determine Independent Signals/1(BattVltgCorrlnOk)
  [BattVltgSwd1CorrlnOk] -> Determine Independent Signals/2(BattVltgSwd1CorrlnOk)
  [BattVltgSwd2CorrlnOk] -> Determine Independent Signals/3(BattVltgSwd2CorrlnOk)
  DiagcStsIvtr1Inactv/1 -> Determine Independent Signals/4(DiagcStsIvtr1Inactv)
  DiagcStsIvtr2Inactv/1 -> Determine Independent Signals/5(DiagcStsIvtr2Inactv)
  Determine Independent Signals/1(BattVltgPassed) -> [BattVltgPassed]
  Determine Independent Signals/2(BattVltgSwd1Passed) -> [BattVltgSwd1Passed]
  Determine Independent Signals/3(BattVltgSwd2Passed) -> [BattVltgSwd2Passed]
  Determine Independent Signals/4(BattVltgCorrlnIdptSig) -> BattVltgCorrlnIdptSig/1
  [BattVltgCorrlnOk] -> Determine Correlation Status/1(BattVltgCorrlnOk)
  [BattVltgPassed] -> Determine Correlation Status/2(BattVltgPassed)
  [BattVltgSwd1CorrlnOk] -> Determine Correlation Status/3(BattVltgSwd1CorrlnOk)
  [BattVltgSwd1Passed] -> Determine Correlation Status/4(BattVltgSwd1Passed)
  [BattVltgSwd2CorrlnOk] -> Determine Correlation Status/5(BattVltgSwd2CorrlnOk)
  [BattVltgSwd2Passed] -> Determine Correlation Status/6(BattVltgSwd2Passed)
  Determine Correlation Status/1(BattVltgCorrlnSts) -> BattVltgCorrlnSts/1
  Instantaneous Correlation/4(SwdVltgLimd) -> SwdVltgLimd/1
  BattVltgAdcFaild/1 -> Instantaneous Correlation/4(BattVltgAdcFaild)
  BattVltgSwd1AdcFaild/1 -> Instantaneous Correlation/5(BattVltgSwd1AdcFaild)
  BattVltgSwd2AdcFaild/1 -> Instantaneous Correlation/6(BattVltgSwd2AdcFaild)
  Determine Correlation Status/2(DftBrdgVltgActv) -> DftBrdgVltgActv/1
  Instantaneous Correlation/3(BattVltgSwd2CorrlnOk) -> [BattVltgSwd2CorrlnOk]

== system ES259A_BattVltgCorrln/BattVltgCorrln/BattVltgCorrlnPer1/Battery Voltage Diagnostics/Copyright1 ==

== system ES259A_BattVltgCorrln/BattVltgCorrln/BattVltgCorrlnPer1/Battery Voltage Diagnostics/Inhibition Off ==
  note: Outside Operational Voltage Range (No Assist)						0x0B0
      | 	Under Minimum Battery Voltage
      | Extended Voltage Range, Low Voltage (Extended Performance)			0x0B1
      | 	Low Battery Voltage
      | Outside Operational Voltage Range (No Assist)						0x0B5
      | 	Over Maximum Battery Voltage
  BattVltg : Inport
  Action Port : ActionPort  ActionType=then
  BattVltg < UnderVltg : Subsystem  RequirementInfo={} %GIDa_27210ad8_0da4_4b7d_ad34_47372fdcd46e  TreatAsAtomicUnit=on
  BattVltg > OverVltg : Subsystem  RequirementInfo={} %GIDa_f678b1bc_f111_4fcf_b4f9_eeaa0479fbc9  TreatAsAtomicUnit=on
  Constant : Constant  Value=BattVltgCorrlnBattLoVltg
  Constant1 : Constant  Value=BattVltgCorrlnBattOverVltg
  Constant2 : Constant  Value=BattVltgCorrlnBattUnderVltg
  Copyright1 : Subsystem  Description=|  mask(Copyright Information){none=on}
      | Copyright info block.                                               
      |                                                                     
      | Place copyright information at the top of every subsystem in design.
      mask prompts: none "No parameters"
      mask help: Place copyright information at the top of every subsystem in design.
      mask Display:
      | NxtrConf = 'Nexteer Confidential';
      | 
      | sys = bdroot; %handle for the current model ("system")
      | first = get_param(sys,'Created');
      | if(isempty(first))
      |     first = datestr(now,'yyyy');
      | else
      |     first = first(end-3:end);  %year is last four digits
      | end
      | 
      | last = get_param(sys,'LastModifiedDate');
      | if isempty(last)
      |     last = datestr(now,'yyyy');
      | else
      |     last = last(end-3:end);
      | end
      | 
      | if strcmp(first,last)
      |     fprintf('%s\nCopyright  %s Nexteer',NxtrConf,first);
      | else
      |     fprintf('%s\n%s%s-%s Nexteer',NxtrConf,char(169),first,last);
      | end
  If : If  NumInputs=4  IfExpression=u1 > u2  ElseIfExpressions=((u1 < u3) & (u1 >= u4)), u1 < u4
  LowVltg <= Batt <= OverVltg : Subsystem  RequirementInfo={} %GIDa_9c974e7b_bca6_4d23_a789_0c8532e06c78  TreatAsAtomicUnit=on
  UnderVltg <= BattVltg < LowVltg : Subsystem  RequirementInfo={} %GIDa_4ff1a3e6_7cb5_4c5b_8a30_2a844fcdd7f9  TreatAsAtomicUnit=on
  wires:
  Constant1/1 -> If/2
  Constant2/1 -> If/4
  Constant/1 -> If/3
  If/1 -> BattVltg > OverVltg/Action
  If/2 -> UnderVltg <= BattVltg < LowVltg/Action
  If/3 -> BattVltg < UnderVltg/Action
  If/4 -> LowVltg <= Batt <= OverVltg/Action
  BattVltg/1 -> UnderVltg <= BattVltg < LowVltg/1(BattVltg), LowVltg <= Batt <= OverVltg/1(BattVltg), If/1

== system ES259A_BattVltgCorrln/BattVltgCorrln/BattVltgCorrlnPer1/Battery Voltage Diagnostics/Inhibition On ==
  Action Port : ActionPort  ActionType=else
  Copyright1 : Subsystem  Description=|  mask(Copyright Information){none=on}
      | Copyright info block.                                               
      |                                                                     
      | Place copyright information at the top of every subsystem in design.
      mask prompts: none "No parameters"
      mask help: Place copyright information at the top of every subsystem in design.
      mask Display:
      | NxtrConf = 'Nexteer Confidential';
      | 
      | sys = bdroot; %handle for the current model ("system")
      | first = get_param(sys,'Created');
      | if(isempty(first))
      |     first = datestr(now,'yyyy');
      | else
      |     first = first(end-3:end);  %year is last four digits
      | end
      | 
      | last = get_param(sys,'LastModifiedDate');
      | if isempty(last)
      |     last = datestr(now,'yyyy');
      | else
      |     last = last(end-3:end);
      | end
      | 
      | if strcmp(first,last)
      |     fprintf('%s\nCopyright  %s Nexteer',NxtrConf,first);
      | else
      |     fprintf('%s\n%s%s-%s Nexteer',NxtrConf,char(169),first,last);
      | end

== system ES259A_BattVltgCorrln/BattVltgCorrln/BattVltgCorrlnPer1/Disable State/Copyright1 ==

== system ES259A_BattVltgCorrln/BattVltgCorrln/BattVltgCorrlnPer1/WarmInit or Enable/Copyright1 ==

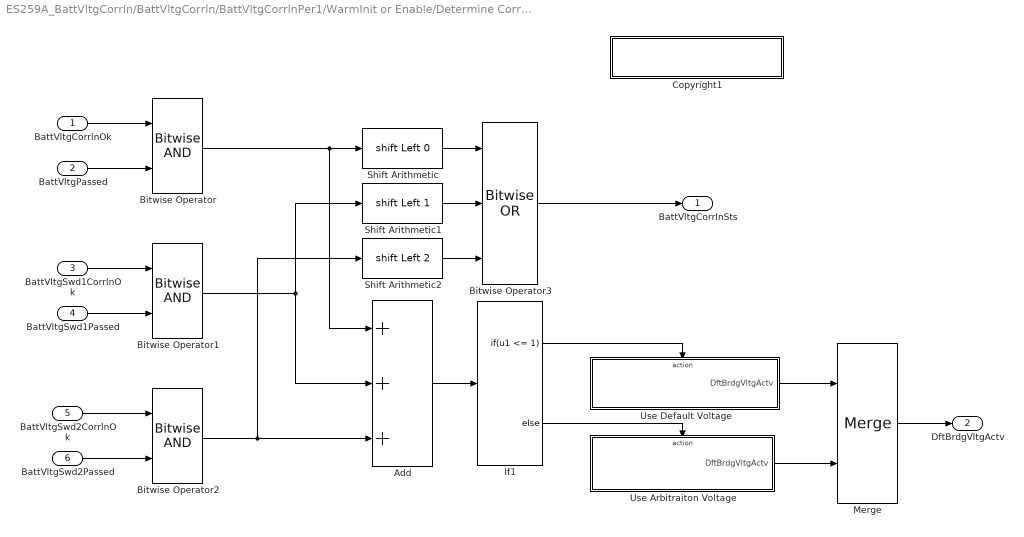
== system ES259A_BattVltgCorrln/BattVltgCorrln/BattVltgCorrlnPer1/WarmInit or Enable/Determine Correlation Status ==
  BattVltgCorrlnOk : Inport
  BattVltgPassed : Inport  Port=2
  BattVltgSwd1CorrlnOk : Inport  Port=3
  BattVltgSwd1Passed : Inport  Port=4
  BattVltgSwd2CorrlnOk : Inport  Port=5
  BattVltgSwd2Passed : Inport  Port=6
  Add : Sum  Inputs=+++
  Bitwise Operator : simulink/Logic and Bit Operations/Bitwise Operator  logicop=AND  UseBitMask=off  NumInputPorts=2  BitMask=bin2dec('11011001')  BitMaskRealWorld=Stored Integer
  Bitwise Operator1 : simulink/Logic and Bit Operations/Bitwise Operator  logicop=AND  UseBitMask=off  NumInputPorts=2  BitMask=bin2dec('11011001')  BitMaskRealWorld=Stored Integer
  Bitwise Operator2 : simulink/Logic and Bit Operations/Bitwise Operator  logicop=AND  UseBitMask=off  NumInputPorts=2  BitMask=bin2dec('11011001')  BitMaskRealWorld=Stored Integer
  Bitwise Operator3 : simulink/Logic and Bit Operations/Bitwise Operator  logicop=OR  UseBitMask=off  NumInputPorts=3  BitMask=bin2dec('11011001')  BitMaskRealWorld=Stored Integer
  Copyright1 : Subsystem  Description=|  mask(Copyright Information){none=on}
      | Copyright info block.                                               
      |                                                                     
      | Place copyright information at the top of every subsystem in design.
      mask prompts: none "No parameters"
      mask help: Place copyright information at the top of every subsystem in design.
      mask Display:
      | NxtrConf = 'Nexteer Confidential';
      | 
      | sys = bdroot; %handle for the current model ("system")
      | first = get_param(sys,'Created');
      | if(isempty(first))
      |     first = datestr(now,'yyyy');
      | else
      |     first = first(end-3:end);  %year is last four digits
      | end
      | 
      | last = get_param(sys,'LastModifiedDate');
      | if isempty(last)
      |     last = datestr(now,'yyyy');
      | else
      |     last = last(end-3:end);
      | end
      | 
      | if strcmp(first,last)
      |     fprintf('%s\nCopyright  %s Nexteer',NxtrConf,first);
      | else
      |     fprintf('%s\n%s%s-%s Nexteer',NxtrConf,char(169),first,last);
      | end
  If1 : If  IfExpression=u1 <= 1
  Merge : Merge
  Shift Arithmetic : ArithShift  BitShiftDirection=Left
  Shift Arithmetic1 : ArithShift  BitShiftNumber=1  BitShiftDirection=Left
  Shift Arithmetic2 : ArithShift  BitShiftNumber=2  BitShiftDirection=Left
  Use Arbitraiton Voltage : Subsystem  TreatAsAtomicUnit=on
  Use Default Voltage : Subsystem  TreatAsAtomicUnit=on
  BattVltgCorrlnSts : Outport
  DftBrdgVltgActv : Outport  Port=2
  wires:
  BattVltgPassed/1 -> Bitwise Operator/2
  BattVltgCorrlnOk/1 -> Bitwise Operator/1
  BattVltgSwd1Passed/1 -> Bitwise Operator1/2
  BattVltgSwd1CorrlnOk/1 -> Bitwise Operator1/1
  BattVltgSwd2Passed/1 -> Bitwise Operator2/2
  BattVltgSwd2CorrlnOk/1 -> Bitwise Operator2/1
  If1/1 -> Use Default Voltage/Action
  If1/2 -> Use Arbitraiton Voltage/Action
  Use Default Voltage/1(DftBrdgVltgActv) -> Merge/1
  Use Arbitraiton Voltage/1(DftBrdgVltgActv) -> Merge/2
  Merge/1 -> DftBrdgVltgActv/1
  Add/1 -> If1/1
  Bitwise Operator/1 -> Add/1, Shift Arithmetic/1
  Bitwise Operator1/1 -> Add/2, Shift Arithmetic1/1
  Bitwise Operator2/1 -> Shift Arithmetic2/1, Add/3
  Shift Arithmetic2/1 -> Bitwise Operator3/3
  Shift Arithmetic1/1 -> Bitwise Operator3/2
  Shift Arithmetic/1 -> Bitwise Operator3/1
  Bitwise Operator3/1 -> BattVltgCorrlnSts/1

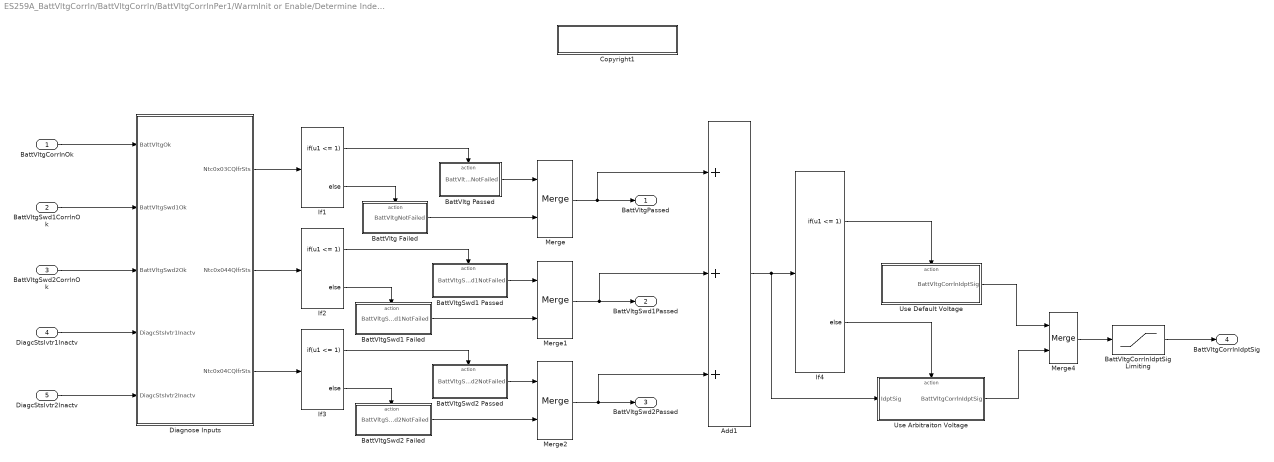
== system ES259A_BattVltgCorrln/BattVltgCorrln/BattVltgCorrlnPer1/WarmInit or Enable/Determine Independent Signals ==
  BattVltgCorrlnOk : Inport
  BattVltgSwd1CorrlnOk : Inport  Port=2  OutDataTypeStr=uint8
  BattVltgSwd2CorrlnOk : Inport  Port=3  OutDataTypeStr=uint8
  DiagcStsIvtr1Inactv : Inport  Port=4
  DiagcStsIvtr2Inactv : Inport  Port=5
  Add1 : Sum  Inputs=+++
  BattVltg Failed : Subsystem
  BattVltg Passed : Subsystem  TreatAsAtomicUnit=on
  BattVltgCorrlnIdptSig Limiting : Saturate  UpperLimit=3  LowerLimit=0
  BattVltgSwd1 Failed : Subsystem
  BattVltgSwd1 Passed : Subsystem  TreatAsAtomicUnit=on
  BattVltgSwd2 Failed : Subsystem
  BattVltgSwd2 Passed : Subsystem  TreatAsAtomicUnit=on
  Copyright1 : Subsystem  Description=|  mask(Copyright Information){none=on}
      | Copyright info block.                                               
      |                                                                     
      | Place copyright information at the top of every subsystem in design.
      mask prompts: none "No parameters"
      mask help: Place copyright information at the top of every subsystem in design.
      mask Display:
      | NxtrConf = 'Nexteer Confidential';
      | 
      | sys = bdroot; %handle for the current model ("system")
      | first = get_param(sys,'Created');
      | if(isempty(first))
      |     first = datestr(now,'yyyy');
      | else
      |     first = first(end-3:end);  %year is last four digits
      | end
      | 
      | last = get_param(sys,'LastModifiedDate');
      | if isempty(last)
      |     last = datestr(now,'yyyy');
      | else
      |     last = last(end-3:end);
      | end
      | 
      | if strcmp(first,last)
      |     fprintf('%s\nCopyright  %s Nexteer',NxtrConf,first);
      | else
      |     fprintf('%s\n%s%s-%s Nexteer',NxtrConf,char(169),first,last);
      | end
  Diagnose Inputs : Subsystem
  If{1..4} (4 alike) : If  IfExpression=u1 <= 1
  Merge{,1..2,4} (4 alike) : Merge
  Use Arbitraiton Voltage : Subsystem  TreatAsAtomicUnit=on
  Use Default Voltage : Subsystem  TreatAsAtomicUnit=on
  BattVltgPassed : Outport
  BattVltgSwd1Passed : Outport  Port=2
  BattVltgSwd2Passed : Outport  Port=3
  BattVltgCorrlnIdptSig : Outport  Port=4
  wires:
  Merge/1 -> BattVltgPassed/1, Add1/1
  Merge1/1 -> BattVltgSwd1Passed/1, Add1/2
  Merge2/1 -> BattVltgSwd2Passed/1, Add1/3
  BattVltgCorrlnOk/1 -> Diagnose Inputs/1(BattVltgOk)
  BattVltgSwd1CorrlnOk/1 -> Diagnose Inputs/2(BattVltgSwd1Ok)
  BattVltgSwd2CorrlnOk/1 -> Diagnose Inputs/3(BattVltgSwd2Ok)
  DiagcStsIvtr1Inactv/1 -> Diagnose Inputs/4(DiagcStsIvtr1Inactv)
  DiagcStsIvtr2Inactv/1 -> Diagnose Inputs/5(DiagcStsIvtr2Inactv)
  Diagnose Inputs/2(Ntc0x044QlfrSts) -> If2/1
  Diagnose Inputs/1(Ntc0x03CQlfrSts) -> If1/1
  Diagnose Inputs/3(Ntc0x04CQlfrSts) -> If3/1
  If1/2 -> BattVltg Failed/Action
  If1/1 -> BattVltg Passed/Action
  BattVltg Failed/1(BattVltgNotFailed) -> Merge/2
  BattVltg Passed/1(BattVltgNotFailed) -> Merge/1
  If2/2 -> BattVltgSwd1 Failed/Action
  If2/1 -> BattVltgSwd1 Passed/Action
  BattVltgSwd1 Failed/1(BattVltgSwd1NotFailed) -> Merge1/2
  BattVltgSwd1 Passed/1(BattVltgSwd1NotFailed) -> Merge1/1
  If3/2 -> BattVltgSwd2 Failed/Action
  If3/1 -> BattVltgSwd2 Passed/Action
  BattVltgSwd2 Failed/1(BattVltgSwd2NotFailed) -> Merge2/2
  BattVltgSwd2 Passed/1(BattVltgSwd2NotFailed) -> Merge2/1
  If4/2 -> Use Arbitraiton Voltage/Action
  BattVltgCorrlnIdptSig Limiting/1 -> BattVltgCorrlnIdptSig/1
  Add1/1 -> Use Arbitraiton Voltage/1(IdptSig), If4/1
  Use Default Voltage/1(BattVltgCorrlnIdptSig) -> Merge4/1
  Use Arbitraiton Voltage/1(BattVltgCorrlnIdptSig) -> Merge4/2
  Merge4/1 -> BattVltgCorrlnIdptSig Limiting/1
  If4/1 -> Use Default Voltage/Action

== system ES259A_BattVltgCorrln/BattVltgCorrln/BattVltgCorrlnPer1/WarmInit or Enable/Instantaneous Correlation ==
  BattVltg : Inport
  BattVltgSwd1 : Inport  Port=2
  BattVltgSwd2 : Inport  Port=3
  BattVltgAdcFaild : Inport  Port=4
  BattVltgSwd1AdcFaild : Inport  Port=5
  BattVltgSwd2AdcFaild : Inport  Port=6
  Bitwise Operator : simulink/Logic and Bit Operations/Bitwise Operator  logicop=AND  UseBitMask=off  NumInputPorts=2  BitMask=bin2dec('11011001')  BitMaskRealWorld=Stored Integer
  Bitwise Operator1 : simulink/Logic and Bit Operations/Bitwise Operator  logicop=AND  UseBitMask=off  NumInputPorts=2  BitMask=bin2dec('11011001')  BitMaskRealWorld=Stored Integer
  Bitwise Operator2 : simulink/Logic and Bit Operations/Bitwise Operator  logicop=AND  UseBitMask=off  NumInputPorts=2  BitMask=bin2dec('11011001')  BitMaskRealWorld=Stored Integer
  Copyright1 : Subsystem  Description=|  mask(Copyright Information){none=on}
      | Copyright info block.                                               
      |                                                                     
      | Place copyright information at the top of every subsystem in design.
      mask prompts: none "No parameters"
      mask help: Place copyright information at the top of every subsystem in design.
      mask Display:
      | NxtrConf = 'Nexteer Confidential';
      | 
      | sys = bdroot; %handle for the current model ("system")
      | first = get_param(sys,'Created');
      | if(isempty(first))
      |     first = datestr(now,'yyyy');
      | else
      |     first = first(end-3:end);  %year is last four digits
      | end
      | 
      | last = get_param(sys,'LastModifiedDate');
      | if isempty(last)
      |     last = datestr(now,'yyyy');
      | else
      |     last = last(end-3:end);
      | end
      | 
      | if strcmp(first,last)
      |     fprintf('%s\nCopyright  %s Nexteer',NxtrConf,first);
      | else
      |     fprintf('%s\n%s%s-%s Nexteer',NxtrConf,char(169),first,last);
      | end
  Correlation Check : Subsystem
  Range Check : Subsystem  RequirementInfo="{'linktype_rmi_doors' '0000cf46 (/ESG Group/FDD Module Requirements/EA4 Specific/ES259A_BattVltgCorrln)' '#ES259A_202' 'true' 'REQ:  ES259A_202' '' ; 'linktype_rmi_doors' '0000cf46 (/ESG Group/FDD Module Requirements/EA4 Specific/ES259A_BattVltgCorrln)' '#ES259A_217' 'true' 'REQ:  ES259A_217' '' ; 'linktype_rmi_doors' '0000cf46 (/ESG Group/FDD Module Requirements/EA4 Specific/ES259A_BattVltgCorrln)' '#ES259A_221' 'true' 'REQ:  ES259A_221' '' } %GIDa_2b173e7d_e60e_4bdc_9f38_bb3a66a6be82"
  BattVltgCorrlnOk : Outport
  BattVltgSwd1CorrlnOk : Outport  Port=2
  BattVltgSwd2CorrlnOk : Outport  Port=3
  SwdVltgLimd : Outport  RequirementInfo={} %GIDa_cf15afd8_a2d9_431a_a2fb_de887df9be9e  Port=4
  wires:
  BattVltg/1 -> Correlation Check/1(BattVltg), Range Check/1(BattVltg)
  BattVltgSwd1/1 -> Range Check/2(BattVltgSwd1), Correlation Check/2(BattVltgSwd1)
  BattVltgAdcFaild/1 -> Correlation Check/4(BattVltgAdcFaild)
  BattVltgSwd1AdcFaild/1 -> Correlation Check/5(BattVltgSwd1AdcFaild)
  BattVltgSwd2AdcFaild/1 -> Correlation Check/6(BattVltgSwd2AdcFaild)
  Correlation Check/4(SwdVltgLimd) -> SwdVltgLimd/1
  BattVltgSwd2/1 -> Correlation Check/3(BattVltgSwd2), Range Check/3(BattVltgSwd2)
  Range Check/1(BattVltgRngOk) -> Bitwise Operator/1
  Correlation Check/3(BattVltgSwd2CorrlnOk) -> Bitwise Operator2/2
  Correlation Check/1(BattVltgCorrlnOk) -> Bitwise Operator/2
  Correlation Check/2(BattVltgSwd1CorrlnOk) -> Bitwise Operator1/2
  Range Check/3(BattVltgSwd2RngOk) -> Bitwise Operator2/1
  Bitwise Operator/1 -> BattVltgCorrlnOk/1
  Bitwise Operator1/1 -> BattVltgSwd1CorrlnOk/1
  Bitwise Operator2/1 -> BattVltgSwd2CorrlnOk/1
  Range Check/2(BattVltgSwd1RngOk) -> Bitwise Operator1/1
